simulink model "lab1simulink"  (R2025a)
settings: Solver=VariableStepAuto  StartTime=0.0  StopTime=50  RelTol=1e-3
undefined symbols (not defined in the file): C, L, R
settings Model: Creator=sunzi  LastModifiedBy=sunzi

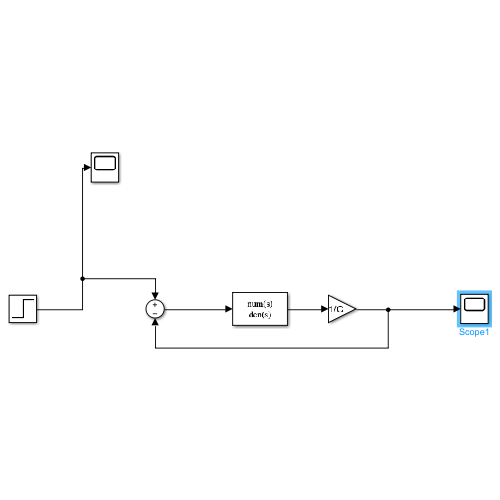
[thumbnail: Simulink's stored preview of the top-level diagram]
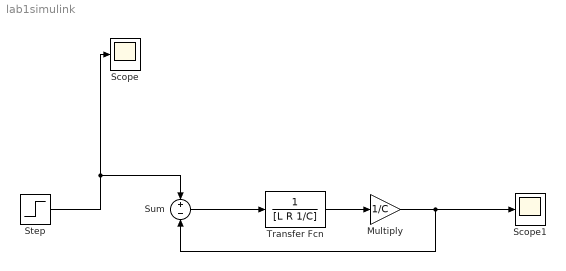
== system lab1simulink ==
  Multiply : Gain  Gain=1/C
  Scope : Scope
      settings: ActiveDisplayYMinimum=-0.12499999999999997  ActiveDisplayYMaximum=1.125
  Scope1 : Scope
      settings: ActiveDisplayYMinimum=-0.0798561568314865  ActiveDisplayYMaximum=0.71870541148337863
  Step : Step  SampleTime=0
  Sum : Sum  Inputs=+-
  Transfer Fcn : TransferFcn  Denominator=[L R 1/C]
  wires:
  Step/1 -> Scope/1, Sum/1
  Sum/1 -> Transfer Fcn/1
  Transfer Fcn/1 -> Multiply/1
  Multiply/1 -> Scope1/1, Sum/2
